simulink model "TestQ"  (R2015b)
settings: Solver=VariableStepAuto  StartTime=0.0  StopTime=120  MaxStep=0.001  RelTol=1e-3
InitFcn:
  | clear
  | load tfwt_00_run_01.mat
  | flog = logOriginal
  | flog.vehicle_attitude.time = flog.vehicle_attitude.time - flog.att_pos_mocap.time(1);
  | flog.sensor_combined.time = flog.sensor_combined.time - flog.att_pos_mocap.time(1);
  | flog.att_pos_mocap.time = flog.att_pos_mocap.time - flog.att_pos_mocap.time(1);
libraries: QuaternionLibrary x2, Px4Library x1
settings Model: Creator=jban039  LastModifiedBy=jban039

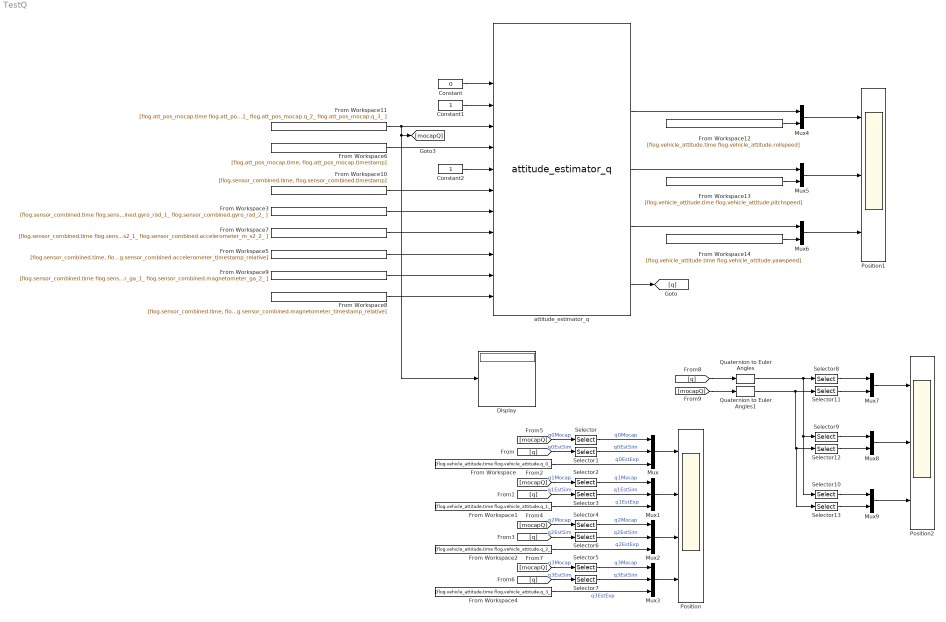
== system TestQ ==
  Constant : Constant  Value=0
  Constant1 : Constant
  Constant2 : Constant
  Display : Display
  From Workspace : FromWorkspace  VariableName=[flog.vehicle_attitude.time flog.vehicle_attitude.q_0_]  SampleTime=0  Interpolate=off  OutputAfterFinalValue=Holding final value
  From Workspace1 : FromWorkspace  VariableName=[flog.vehicle_attitude.time flog.vehicle_attitude.q_1_]  SampleTime=0  Interpolate=off  OutputAfterFinalValue=Holding final value
  From Workspace10 : FromWorkspace  VariableName=[flog.sensor_combined.time, flog.sensor_combined.timestamp]  SampleTime=0  Interpolate=off  OutputAfterFinalValue=Holding final value
  From Workspace11 : FromWorkspace  VariableName=[flog.att_pos_mocap.time flog.att_pos_mocap.q_0_ flog.att_pos_mocap.q_1_ flog.att_pos_mocap.q_2_ flog.att_pos_mocap.q_3_ ]  SampleTime=0  Interpolate=off  OutputAfterFinalValue=Holding final value
  From Workspace12 : FromWorkspace  VariableName=[flog.vehicle_attitude.time flog.vehicle_attitude.rollspeed]  SampleTime=0  Interpolate=off  OutputAfterFinalValue=Holding final value
  From Workspace13 : FromWorkspace  VariableName=[flog.vehicle_attitude.time flog.vehicle_attitude.pitchspeed]  SampleTime=0  Interpolate=off  OutputAfterFinalValue=Holding final value
  From Workspace14 : FromWorkspace  VariableName=[flog.vehicle_attitude.time flog.vehicle_attitude.yawspeed]  SampleTime=0  Interpolate=off  OutputAfterFinalValue=Holding final value
  From Workspace2 : FromWorkspace  VariableName=[flog.vehicle_attitude.time flog.vehicle_attitude.q_2_]  SampleTime=0  Interpolate=off  OutputAfterFinalValue=Holding final value
  From Workspace3 : FromWorkspace  VariableName=[flog.sensor_combined.time flog.sensor_combined.gyro_rad_0_ flog.sensor_combined.gyro_rad_1_ flog.sensor_combined.gyro_rad_2_ ]  SampleTime=0  Interpolate=off  OutputAfterFinalValue=Holding final value
  From Workspace4 : FromWorkspace  VariableName=[flog.vehicle_attitude.time flog.vehicle_attitude.q_3_]  SampleTime=0  Interpolate=off  OutputAfterFinalValue=Holding final value
  From Workspace5 : FromWorkspace  VariableName=[flog.sensor_combined.time, flog.sensor_combined.accelerometer_timestamp_relative]  SampleTime=0  Interpolate=off  OutputAfterFinalValue=Holding final value
  From Workspace6 : FromWorkspace  VariableName=[flog.att_pos_mocap.time, flog.att_pos_mocap.timestamp]  SampleTime=0  Interpolate=off  OutputAfterFinalValue=Holding final value
  From Workspace7 : FromWorkspace  VariableName=[flog.sensor_combined.time flog.sensor_combined.accelerometer_m_s2_0_ flog.sensor_combined.accelerometer_m_s2_1_ flog.sensor_combined.accelerometer_m_s2_2_ ]  SampleTime=0  Interpolate=off  OutputAfterFinalValue=Holding final value
  From Workspace8 : FromWorkspace  VariableName=[flog.sensor_combined.time, flog.sensor_combined.magnetometer_timestamp_relative]  SampleTime=0  Interpolate=off  OutputAfterFinalValue=Holding final value
  From Workspace9 : FromWorkspace  VariableName=[flog.sensor_combined.time flog.sensor_combined.magnetometer_ga_0_ flog.sensor_combined.magnetometer_ga_1_ flog.sensor_combined.magnetometer_ga_2_ ]  SampleTime=0  Interpolate=off  OutputAfterFinalValue=Holding final value
  Mux{,1..3} (4 alike) : Mux  Inputs=3
  Mux{4..9} (6 alike) : Mux  Inputs=2
  Position : Scope  NumInputPorts=4
  Position1 : Scope  NumInputPorts=3
  Position2 : Scope  NumInputPorts=3
  Quaternion to Euler Angles : QuaternionLibrary/Quaternion to Euler Angles
  Quaternion to Euler Angles1 : QuaternionLibrary/Quaternion to Euler Angles
  Selector : Selector  InputPortWidth=4  IndexOptions=Index vector (dialog)  Indices=[1]  OutputSizes=1
  Selector1 : Selector  InputPortWidth=4  IndexOptions=Index vector (dialog)  Indices=[1]  OutputSizes=1
  Selector10 : Selector  InputPortWidth=3  IndexOptions=Index vector (dialog)  Indices=3  OutputSizes=1
  Selector{8..9,11..12} (4 alike) : Selector  InputPortWidth=3  IndexOptions=Index vector (dialog)  Indices=[1]  OutputSizes=1
  Selector13 : Selector  InputPortWidth=3  IndexOptions=Index vector (dialog)  Indices=3  OutputSizes=1
  Selector2 : Selector  InputPortWidth=4  IndexOptions=Index vector (dialog)  Indices=2  OutputSizes=1
  Selector3 : Selector  InputPortWidth=4  IndexOptions=Index vector (dialog)  Indices=2  OutputSizes=1
  Selector4 : Selector  InputPortWidth=4  IndexOptions=Index vector (dialog)  Indices=3  OutputSizes=1
  Selector5 : Selector  InputPortWidth=4  IndexOptions=Index vector (dialog)  Indices=4  OutputSizes=1
  Selector6 : Selector  InputPortWidth=4  IndexOptions=Index vector (dialog)  Indices=3  OutputSizes=1
  Selector7 : Selector  InputPortWidth=4  IndexOptions=Index vector (dialog)  Indices=4  OutputSizes=1
  attitude_estimator_q : Px4Library/attitude_estimator_q  Q_SAMPLING_PERIOD=1/250  ATT_W_ACC=0.200  ATT_W_MAG=0.100  ATT_W_EXT_HDG=0.100  ATT_W_GYRO_BIAS=0.100  ATT_MAG_DECL=0.0  ATT_MAG_DECL_A=1.000  ATT_EXT_HDG_M=2  ATT_ACC_COMP=1.000  ATT_BIAS_MAX=0.050  FW_ARSP_MODE=0
  wires:
  Mux1/1 -> Position/2
  Mux/1 -> Position/1
  Mux2/1 -> Position/3
  attitude_estimator_q/5 -> [q]
  From Workspace/1 -> Mux/3  "q0EstExp"
  Selector1/1 -> Mux/2  "q0EstSim"
  From Workspace11/1 -> attitude_estimator_q/5, Display/1, [mocapQ]
  From Workspace6/1 -> attitude_estimator_q/6
  Constant/1 -> attitude_estimator_q/3
  Selector/1 -> Mux/1  "q0Mocap"
  Constant1/1 -> attitude_estimator_q/4
  From Workspace7/1 -> attitude_estimator_q/10
  From Workspace9/1 -> attitude_estimator_q/12
  From Workspace10/1 -> attitude_estimator_q/8
  Constant2/1 -> attitude_estimator_q/7
  From Workspace3/1 -> attitude_estimator_q/9
  From Workspace1/1 -> Mux1/3  "q1EstExp"
  Selector3/1 -> Mux1/2  "q1EstSim"
  Selector2/1 -> Mux1/1  "q1Mocap"
  From Workspace2/1 -> Mux2/3  "q2EstExp"
  Selector6/1 -> Mux2/2  "q2EstSim"
  Selector4/1 -> Mux2/1  "q2Mocap"
  Mux3/1 -> Position/4
  From Workspace4/1 -> Mux3/3  "q3EstExp"
  Selector7/1 -> Mux3/2  "q3EstSim"
  Selector5/1 -> Mux3/1  "q3Mocap"
  [mocapQ] -> Selector/1  "q0Mocap"
  [q] -> Selector1/1  "q0EstSim"
  [mocapQ] -> Selector2/1  "q1Mocap"
  [q] -> Selector3/1  "q1EstSim"
  [mocapQ] -> Selector4/1  "q2Mocap"
  [q] -> Selector6/1  "q2EstSim"
  [mocapQ] -> Selector5/1  "q3Mocap"
  [q] -> Selector7/1  "q3EstSim"
  From Workspace8/1 -> attitude_estimator_q/13
  From Workspace5/1 -> attitude_estimator_q/11
  Mux4/1 -> Position1/1
  Mux5/1 -> Position1/2
  Mux6/1 -> Position1/3
  attitude_estimator_q/2 -> Mux4/1
  attitude_estimator_q/3 -> Mux5/1
  attitude_estimator_q/4 -> Mux6/1
  From Workspace12/1 -> Mux4/2
  From Workspace13/1 -> Mux5/2
  From Workspace14/1 -> Mux6/2
  Quaternion to Euler Angles/1 -> Selector10/1, Selector9/1, Selector8/1
  Quaternion to Euler Angles1/1 -> Selector13/1, Selector12/1, Selector11/1
  Mux7/1 -> Position2/1
  Mux8/1 -> Position2/2
  Mux9/1 -> Position2/3
  Selector8/1 -> Mux7/1
  Selector11/1 -> Mux7/2
  Selector9/1 -> Mux8/1
  Selector12/1 -> Mux8/2
  Selector13/1 -> Mux9/2
  Selector10/1 -> Mux9/1
  [mocapQ] -> Quaternion to Euler Angles1/1
  [q] -> Quaternion to Euler Angles/1
